simulink model "DC_Motor_CoastMode"  (R2018a)
settings: Solver=VariableStepAuto  StartTime=0.0  StopTime=10  RelTol=1e-3
PreLoadFcn:
  | modelDir = fileparts(get_param(bdroot, 'FileName'));
  | addpath(fullfile(modelDir,'Parameters'));
  | addpath(fullfile(modelDir,'subsystems'));
  | 
  | Parameters_Model
  | Parameters_Simulation
  | Parameters_Controller
InitFcn:
  | Parameters_Model
  | Parameters_Simulation
  | Parameters_Controller
undefined symbols (not defined in the file): B, dTheta0, I0, J, Ke, Kt, L, R, theta0
settings Model: Creator=Thomas  LastModifiedBy=Thomas

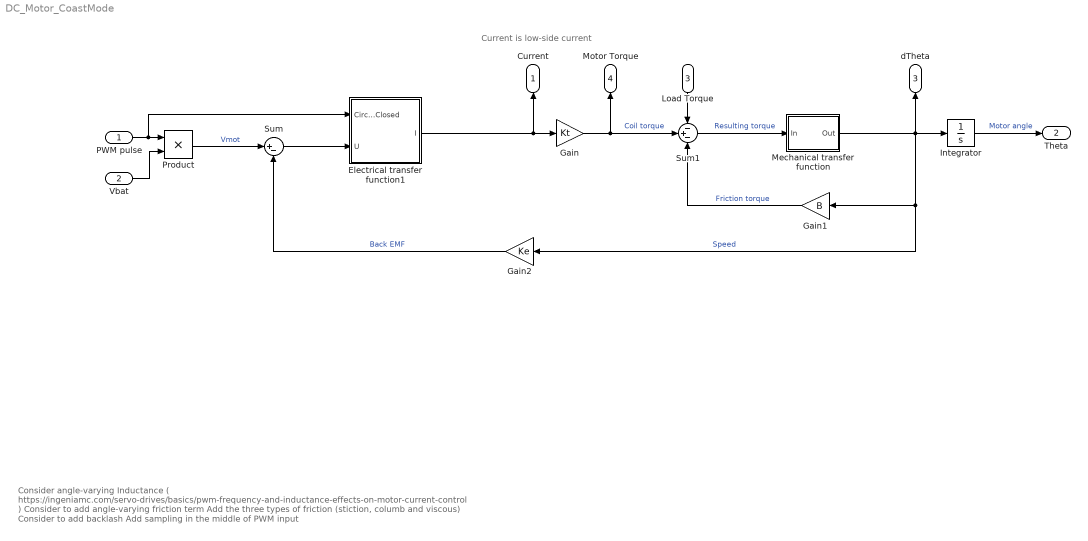
== system DC_Motor_CoastMode ==
  note: Current is low-side current
  note: Consider angle-varying Inductance ( https://ingeniamc.com/servo-drives/basics/pwm-frequency-and-inductance-effects-on-motor-current-control )
      | Consider to add angle-varying friction term
      | Add the three types of friction (stiction, columb and viscous)
      | Consider to add backlash
      | Add sampling in the middle of PWM input
  PWM pulse : Inport  OutDataTypeStr=boolean
  Vbat : Inport  Port=2  OutDataTypeStr=double
  Load Torque : Inport  Port=3
  Electrical transfer function1 : Subsystem
  Gain : Gain  Gain=Kt
  Gain1 : Gain  Gain=B
  Gain2 : Gain  Gain=Ke
  Integrator : Integrator  InitialCondition=theta0
  Mechanical transfer function : Subsystem
  Product : Product
  Sum : Sum  Inputs=|+-
  Sum1 : Sum  Inputs=-+-
  Current : Outport
  Theta : Outport  Port=2
  dTheta : Outport  Port=3
  Motor Torque : Outport  Port=4
  wires:
  Vbat/1 -> Product/2
  Product/1 -> Sum/1  "Vmot"
  Electrical transfer function1/1(I) -> Current/1, Gain/1
  Sum/1 -> Electrical transfer function1/2(U)
  Gain2/1 -> Sum/2  "Back EMF"
  Gain/1 -> Sum1/2, Motor Torque/1  "Coil torque"
  Load Torque/1 -> Sum1/1
  Sum1/1 -> Mechanical transfer function/1(In)  "Resulting torque"
  Mechanical transfer function/1(Out) -> Gain2/1, Gain1/1, Integrator/1, dTheta/1  "Speed"
  Gain1/1 -> Sum1/3  "Friction torque"
  Integrator/1 -> Theta/1  "Motor angle"
  PWM pulse/1 -> Electrical transfer function1/1(CircuitClosed), Product/1

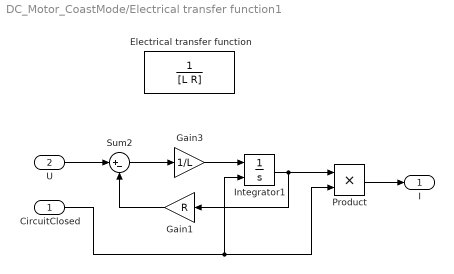
== system DC_Motor_CoastMode/Electrical transfer function1 ==
  CircuitClosed : Inport
  U : Inport  Port=2
  Electrical transfer function : TransferFcn  Denominator=[L R]
  Gain1 : Gain  Gain=R
  Gain3 : Gain  Gain=1/L
  Integrator1 : Integrator  ExternalReset=either  InitialCondition=I0
  Product : Product
  Sum2 : Sum  Inputs=|+-
  I : Outport
  wires:
  U/1 -> Sum2/1
  Gain3/1 -> Integrator1/1
  Gain1/1 -> Sum2/2
  Sum2/1 -> Gain3/1
  Integrator1/1 -> Product/1, Gain1/1
  CircuitClosed/1 -> Product/2, Integrator1/2
  Product/1 -> I/1

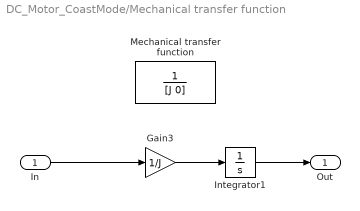
== system DC_Motor_CoastMode/Mechanical transfer function ==
  In : Inport
  Gain3 : Gain  Gain=1/J
  Integrator1 : Integrator  InitialCondition=dTheta0
  Mechanical transfer function : TransferFcn  Denominator=[J 0]
  Out : Outport
  wires:
  Gain3/1 -> Integrator1/1
  In/1 -> Gain3/1
  Integrator1/1 -> Out/1
